simulink model "tp3"  (R2015b)
settings: Solver=VariableStepAuto  StartTime=0.0  StopTime=10  RelTol=1e-3
undefined symbols (not defined in the file or in its folder): tau1, tau2
settings Model: Creator=max.sonzogni  LastModifiedBy=max.sonzogni

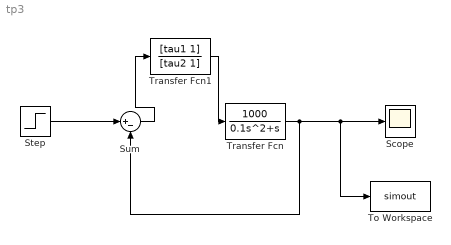
== system tp3 ==
  Scope : Scope
  Step : Step  SampleTime=0
  Sum : Sum  Inputs=|+-
  To Workspace : ToWorkspace  VariableName=simout  SaveFormat=Timeseries  SampleTime=-1
  Transfer Fcn : TransferFcn  Numerator=[1000]  Denominator=[0.1 1 0]
  Transfer Fcn1 : TransferFcn  Numerator=[tau1 1]  Denominator=[tau2 1]
  wires:
  Step/1 -> Sum/1
  Transfer Fcn/1 -> Scope/1, To Workspace/1, Sum/2
  Transfer Fcn1/1 -> Transfer Fcn/1
  Sum/1 -> Transfer Fcn1/1
